simulink model "CryoDetMultiChan_CMB"  (R2016b)
settings: Solver=ode45  StartTime=0.0  StopTime=1000e-6  MaxStep=Tclk/4  RelTol=1e-3
values from neighbouring files (symbols this model uses):
  ds_axi = 16    [setupCryoFPGA_CMB.m]
  Fclk = Fadc    (= 307200000)    [setupCryoFPGA.m]    (also in setupCryoFPGA_CMB.m; setupCryoFPGAorig.m = 312500000)
  notch = tf( [1 a*wNotch/Q wNotch^2], [1 wNotch/Q wNotch^2])    [setupCryoFPGA.m]    (also in setupCryoFPGA_CMB.m; setupCryoFPGAorig.m)
  notch2 = tf( [1 a*wNotch/Q wNotch^2], [1 wNotch/Q wNotch^2])    [setupCryoFPGA.m]    (also in setupCryoFPGA_CMB.m; setupCryoFPGAorig.m)
  notch3 = tf( [1 a*wNotch/Q wNotch^2], [1 wNotch/Q wNotch^2])    [setupCryoFPGA.m]    (also in setupCryoFPGA_CMB.m; setupCryoFPGAorig.m)
  notch4 = tf( [1 a*wNotch/Q wNotch^2], [1 wNotch/Q wNotch^2])    [setupCryoFPGA.m]    (also in setupCryoFPGA_CMB.m; setupCryoFPGAorig.m)
  Tclk = 1/Fclk    (= 3.25520833333e-09)    [setupCryoFPGA.m]    (also in setupCryoFPGA_CMB.m; setupCryoFPGAorig.m = 3.2e-09)
  Ts = 1/Fadc    (= 3.25520833333e-09)    [setupCryoFPGA.m]    (also in setupCryoFPGA_CMB.m; setupCryoFPGAorig.m = 3.2e-09)
undefined symbols (not defined in the file or in its folder): AXI4, i, Lite, xlipgetpartsetting
libraries: xbsIndex_r4 x2077, CryoDetLib x32, hdlsllib x6, simulink x3
(part 6 of 15)

== system CryoDetMultiChan_CMB/DspCore/Status & Debug/DownSample ==
  note: DownSample with rate change given by Naxi
  In : Inport
  Down Sample : xbsIndex_r4/Down Sample  sample_ratio=Naxi  sample_phase="Last Value of Frame  (most efficient)"  en=off  rst=off  latency=1  dbl_ovrd=off  block_type=dsamp
  Register : xbsIndex_r4/Register  init=0  rst=off  en=off  dbl_ovrd=off  block_type=register
  Register1 : xbsIndex_r4/Register  init=0  rst=off  en=off  dbl_ovrd=off  block_type=register
  Out : Outport
  wires:
  Register1/1 -> Out/1
  Down Sample/1 -> Register/1
  In/1 -> Down Sample/1
  Register/1 -> Register1/1

== system CryoDetMultiChan_CMB/DspCore/Status & Debug/DownSample1 ==
  note: DownSample with rate change given by Naxi
  In : Inport
  Down Sample : xbsIndex_r4/Down Sample  sample_ratio=Naxi  sample_phase="Last Value of Frame  (most efficient)"  en=off  rst=off  latency=1  dbl_ovrd=off  block_type=dsamp
  Register : xbsIndex_r4/Register  init=0  rst=off  en=off  dbl_ovrd=off  block_type=register
  Register1 : xbsIndex_r4/Register  init=0  rst=off  en=off  dbl_ovrd=off  block_type=register
  Out : Outport
  wires:
  Register1/1 -> Out/1
  Down Sample/1 -> Register/1
  In/1 -> Down Sample/1
  Register/1 -> Register1/1

== system CryoDetMultiChan_CMB/DspCore/Status & Debug/DownSample10 ==
  note: DownSample with rate change given by Naxi
  In : Inport
  Down Sample : xbsIndex_r4/Down Sample  sample_ratio=Naxi  sample_phase="Last Value of Frame  (most efficient)"  en=off  rst=off  latency=1  dbl_ovrd=off  block_type=dsamp
  Register : xbsIndex_r4/Register  init=0  rst=off  en=off  dbl_ovrd=off  block_type=register
  Register1 : xbsIndex_r4/Register  init=0  rst=off  en=off  dbl_ovrd=off  block_type=register
  Out : Outport
  wires:
  Register1/1 -> Out/1
  Down Sample/1 -> Register/1
  In/1 -> Down Sample/1
  Register/1 -> Register1/1

== system CryoDetMultiChan_CMB/DspCore/Status & Debug/DownSample11 ==
  note: DownSample with rate change given by Naxi
  In : Inport
  Down Sample : xbsIndex_r4/Down Sample  sample_ratio=Naxi  sample_phase="Last Value of Frame  (most efficient)"  en=off  rst=off  latency=1  dbl_ovrd=off  block_type=dsamp
  Register : xbsIndex_r4/Register  init=0  rst=off  en=off  dbl_ovrd=off  block_type=register
  Register1 : xbsIndex_r4/Register  init=0  rst=off  en=off  dbl_ovrd=off  block_type=register
  Out : Outport
  wires:
  Register1/1 -> Out/1
  Down Sample/1 -> Register/1
  In/1 -> Down Sample/1
  Register/1 -> Register1/1

== system CryoDetMultiChan_CMB/DspCore/Status & Debug/DownSample12 ==
  note: DownSample with rate change given by Naxi
  In : Inport
  Down Sample : xbsIndex_r4/Down Sample  sample_ratio=Naxi  sample_phase="Last Value of Frame  (most efficient)"  en=off  rst=off  latency=1  dbl_ovrd=off  block_type=dsamp
  Register : xbsIndex_r4/Register  init=0  rst=off  en=off  dbl_ovrd=off  block_type=register
  Register1 : xbsIndex_r4/Register  init=0  rst=off  en=off  dbl_ovrd=off  block_type=register
  Out : Outport
  wires:
  Register1/1 -> Out/1
  Down Sample/1 -> Register/1
  In/1 -> Down Sample/1
  Register/1 -> Register1/1

== system CryoDetMultiChan_CMB/DspCore/Status & Debug/DownSample13 ==
  note: DownSample with rate change given by Naxi
  In : Inport
  Down Sample : xbsIndex_r4/Down Sample  sample_ratio=Naxi  sample_phase="Last Value of Frame  (most efficient)"  en=off  rst=off  latency=1  dbl_ovrd=off  block_type=dsamp
  Register : xbsIndex_r4/Register  init=0  rst=off  en=off  dbl_ovrd=off  block_type=register
  Register1 : xbsIndex_r4/Register  init=0  rst=off  en=off  dbl_ovrd=off  block_type=register
  Out : Outport
  wires:
  Register1/1 -> Out/1
  Down Sample/1 -> Register/1
  In/1 -> Down Sample/1
  Register/1 -> Register1/1

== system CryoDetMultiChan_CMB/DspCore/Status & Debug/DownSample14 ==
  note: DownSample with rate change given by Naxi
  In : Inport
  Down Sample : xbsIndex_r4/Down Sample  sample_ratio=Naxi  sample_phase="Last Value of Frame  (most efficient)"  en=off  rst=off  latency=1  dbl_ovrd=off  block_type=dsamp
  Register : xbsIndex_r4/Register  init=0  rst=off  en=off  dbl_ovrd=off  block_type=register
  Register1 : xbsIndex_r4/Register  init=0  rst=off  en=off  dbl_ovrd=off  block_type=register
  Out : Outport
  wires:
  Register1/1 -> Out/1
  Down Sample/1 -> Register/1
  In/1 -> Down Sample/1
  Register/1 -> Register1/1

== system CryoDetMultiChan_CMB/DspCore/Status & Debug/DownSample15 ==
  note: DownSample with rate change given by Naxi
  In : Inport
  Down Sample : xbsIndex_r4/Down Sample  sample_ratio=Naxi  sample_phase="Last Value of Frame  (most efficient)"  en=off  rst=off  latency=1  dbl_ovrd=off  block_type=dsamp
  Register : xbsIndex_r4/Register  init=0  rst=off  en=off  dbl_ovrd=off  block_type=register
  Register1 : xbsIndex_r4/Register  init=0  rst=off  en=off  dbl_ovrd=off  block_type=register
  Out : Outport
  wires:
  Register1/1 -> Out/1
  Down Sample/1 -> Register/1
  In/1 -> Down Sample/1
  Register/1 -> Register1/1

== system CryoDetMultiChan_CMB/DspCore/Status & Debug/DownSample16 ==
  note: DownSample with rate change given by Naxi
  In : Inport
  Down Sample : xbsIndex_r4/Down Sample  sample_ratio=Naxi  sample_phase="Last Value of Frame  (most efficient)"  en=off  rst=off  latency=1  dbl_ovrd=off  block_type=dsamp
  Register : xbsIndex_r4/Register  init=0  rst=off  en=off  dbl_ovrd=off  block_type=register
  Register1 : xbsIndex_r4/Register  init=0  rst=off  en=off  dbl_ovrd=off  block_type=register
  Out : Outport
  wires:
  Register1/1 -> Out/1
  Down Sample/1 -> Register/1
  In/1 -> Down Sample/1
  Register/1 -> Register1/1

== system CryoDetMultiChan_CMB/DspCore/Status & Debug/DownSample17 ==
  note: DownSample with rate change given by Naxi
  In : Inport
  Down Sample : xbsIndex_r4/Down Sample  sample_ratio=Naxi  sample_phase="Last Value of Frame  (most efficient)"  en=off  rst=off  latency=1  dbl_ovrd=off  block_type=dsamp
  Register : xbsIndex_r4/Register  init=0  rst=off  en=off  dbl_ovrd=off  block_type=register
  Register1 : xbsIndex_r4/Register  init=0  rst=off  en=off  dbl_ovrd=off  block_type=register
  Out : Outport
  wires:
  Register1/1 -> Out/1
  Down Sample/1 -> Register/1
  In/1 -> Down Sample/1
  Register/1 -> Register1/1

== system CryoDetMultiChan_CMB/DspCore/Status & Debug/DownSample18 ==
  note: DownSample with rate change given by Naxi
  In : Inport
  Down Sample : xbsIndex_r4/Down Sample  sample_ratio=Naxi  sample_phase="Last Value of Frame  (most efficient)"  en=off  rst=off  latency=1  dbl_ovrd=off  block_type=dsamp
  Register : xbsIndex_r4/Register  init=0  rst=off  en=off  dbl_ovrd=off  block_type=register
  Register1 : xbsIndex_r4/Register  init=0  rst=off  en=off  dbl_ovrd=off  block_type=register
  Out : Outport
  wires:
  Register1/1 -> Out/1
  Down Sample/1 -> Register/1
  In/1 -> Down Sample/1
  Register/1 -> Register1/1

== system CryoDetMultiChan_CMB/DspCore/Status & Debug/DownSample19 ==
  note: DownSample with rate change given by Naxi
  In : Inport
  Down Sample : xbsIndex_r4/Down Sample  sample_ratio=Naxi  sample_phase="Last Value of Frame  (most efficient)"  en=off  rst=off  latency=1  dbl_ovrd=off  block_type=dsamp
  Register : xbsIndex_r4/Register  init=0  rst=off  en=off  dbl_ovrd=off  block_type=register
  Register1 : xbsIndex_r4/Register  init=0  rst=off  en=off  dbl_ovrd=off  block_type=register
  Out : Outport
  wires:
  Register1/1 -> Out/1
  Down Sample/1 -> Register/1
  In/1 -> Down Sample/1
  Register/1 -> Register1/1

== system CryoDetMultiChan_CMB/DspCore/Status & Debug/DownSample2 ==
  note: DownSample with rate change given by Naxi
  In : Inport
  Down Sample : xbsIndex_r4/Down Sample  sample_ratio=Naxi  sample_phase="Last Value of Frame  (most efficient)"  en=off  rst=off  latency=1  dbl_ovrd=off  block_type=dsamp
  Register : xbsIndex_r4/Register  init=0  rst=off  en=off  dbl_ovrd=off  block_type=register
  Register1 : xbsIndex_r4/Register  init=0  rst=off  en=off  dbl_ovrd=off  block_type=register
  Out : Outport
  wires:
  Register1/1 -> Out/1
  Down Sample/1 -> Register/1
  In/1 -> Down Sample/1
  Register/1 -> Register1/1

== system CryoDetMultiChan_CMB/DspCore/Status & Debug/DownSample20 ==
  note: DownSample with rate change given by Naxi
  In : Inport
  Down Sample : xbsIndex_r4/Down Sample  sample_ratio=Naxi  sample_phase="Last Value of Frame  (most efficient)"  en=off  rst=off  latency=1  dbl_ovrd=off  block_type=dsamp
  Register : xbsIndex_r4/Register  init=0  rst=off  en=off  dbl_ovrd=off  block_type=register
  Register1 : xbsIndex_r4/Register  init=0  rst=off  en=off  dbl_ovrd=off  block_type=register
  Out : Outport
  wires:
  Register1/1 -> Out/1
  Down Sample/1 -> Register/1
  In/1 -> Down Sample/1
  Register/1 -> Register1/1

== system CryoDetMultiChan_CMB/DspCore/Status & Debug/DownSample21 ==
  note: DownSample with rate change given by Naxi
  In : Inport
  Down Sample : xbsIndex_r4/Down Sample  sample_ratio=Naxi  sample_phase="Last Value of Frame  (most efficient)"  en=off  rst=off  latency=1  dbl_ovrd=off  block_type=dsamp
  Register : xbsIndex_r4/Register  init=0  rst=off  en=off  dbl_ovrd=off  block_type=register
  Register1 : xbsIndex_r4/Register  init=0  rst=off  en=off  dbl_ovrd=off  block_type=register
  Out : Outport
  wires:
  Register1/1 -> Out/1
  Down Sample/1 -> Register/1
  In/1 -> Down Sample/1
  Register/1 -> Register1/1

== system CryoDetMultiChan_CMB/DspCore/Status & Debug/DownSample22 ==
  note: DownSample with rate change given by Naxi
  In : Inport
  Down Sample : xbsIndex_r4/Down Sample  sample_ratio=Naxi  sample_phase="Last Value of Frame  (most efficient)"  en=off  rst=off  latency=1  dbl_ovrd=off  block_type=dsamp
  Register : xbsIndex_r4/Register  init=0  rst=off  en=off  dbl_ovrd=off  block_type=register
  Register1 : xbsIndex_r4/Register  init=0  rst=off  en=off  dbl_ovrd=off  block_type=register
  Out : Outport
  wires:
  Register1/1 -> Out/1
  Down Sample/1 -> Register/1
  In/1 -> Down Sample/1
  Register/1 -> Register1/1

== system CryoDetMultiChan_CMB/DspCore/Status & Debug/DownSample23 ==
  note: DownSample with rate change given by Naxi
  In : Inport
  Down Sample : xbsIndex_r4/Down Sample  sample_ratio=Naxi  sample_phase="Last Value of Frame  (most efficient)"  en=off  rst=off  latency=1  dbl_ovrd=off  block_type=dsamp
  Register : xbsIndex_r4/Register  init=0  rst=off  en=off  dbl_ovrd=off  block_type=register
  Register1 : xbsIndex_r4/Register  init=0  rst=off  en=off  dbl_ovrd=off  block_type=register
  Out : Outport
  wires:
  Register1/1 -> Out/1
  Down Sample/1 -> Register/1
  In/1 -> Down Sample/1
  Register/1 -> Register1/1

== system CryoDetMultiChan_CMB/DspCore/Status & Debug/DownSample24 ==
  note: DownSample with rate change given by Naxi
  In : Inport
  Down Sample : xbsIndex_r4/Down Sample  sample_ratio=Naxi  sample_phase="Last Value of Frame  (most efficient)"  en=off  rst=off  latency=1  dbl_ovrd=off  block_type=dsamp
  Register : xbsIndex_r4/Register  init=0  rst=off  en=off  dbl_ovrd=off  block_type=register
  Register1 : xbsIndex_r4/Register  init=0  rst=off  en=off  dbl_ovrd=off  block_type=register
  Out : Outport
  wires:
  Register1/1 -> Out/1
  Down Sample/1 -> Register/1
  In/1 -> Down Sample/1
  Register/1 -> Register1/1

== system CryoDetMultiChan_CMB/DspCore/Status & Debug/DownSample25 ==
  note: DownSample with rate change given by Naxi
  In : Inport
  Down Sample : xbsIndex_r4/Down Sample  sample_ratio=Naxi  sample_phase="Last Value of Frame  (most efficient)"  en=off  rst=off  latency=1  dbl_ovrd=off  block_type=dsamp
  Register : xbsIndex_r4/Register  init=0  rst=off  en=off  dbl_ovrd=off  block_type=register
  Register1 : xbsIndex_r4/Register  init=0  rst=off  en=off  dbl_ovrd=off  block_type=register
  Out : Outport
  wires:
  Register1/1 -> Out/1
  Down Sample/1 -> Register/1
  In/1 -> Down Sample/1
  Register/1 -> Register1/1

== system CryoDetMultiChan_CMB/DspCore/Status & Debug/DownSample26 ==
  note: DownSample with rate change given by Naxi
  In : Inport
  Down Sample : xbsIndex_r4/Down Sample  sample_ratio=Naxi  sample_phase="Last Value of Frame  (most efficient)"  en=off  rst=off  latency=1  dbl_ovrd=off  block_type=dsamp
  Register : xbsIndex_r4/Register  init=0  rst=off  en=off  dbl_ovrd=off  block_type=register
  Register1 : xbsIndex_r4/Register  init=0  rst=off  en=off  dbl_ovrd=off  block_type=register
  Out : Outport
  wires:
  Register1/1 -> Out/1
  Down Sample/1 -> Register/1
  In/1 -> Down Sample/1
  Register/1 -> Register1/1

== system CryoDetMultiChan_CMB/DspCore/Status & Debug/DownSample27 ==
  note: DownSample with rate change given by Naxi
  In : Inport
  Down Sample : xbsIndex_r4/Down Sample  sample_ratio=Naxi  sample_phase="Last Value of Frame  (most efficient)"  en=off  rst=off  latency=1  dbl_ovrd=off  block_type=dsamp
  Register : xbsIndex_r4/Register  init=0  rst=off  en=off  dbl_ovrd=off  block_type=register
  Register1 : xbsIndex_r4/Register  init=0  rst=off  en=off  dbl_ovrd=off  block_type=register
  Out : Outport
  wires:
  Register1/1 -> Out/1
  Down Sample/1 -> Register/1
  In/1 -> Down Sample/1
  Register/1 -> Register1/1

== system CryoDetMultiChan_CMB/DspCore/Status & Debug/DownSample28 ==
  note: DownSample with rate change given by Naxi
  In : Inport
  Down Sample : xbsIndex_r4/Down Sample  sample_ratio=Naxi  sample_phase="Last Value of Frame  (most efficient)"  en=off  rst=off  latency=1  dbl_ovrd=off  block_type=dsamp
  Register : xbsIndex_r4/Register  init=0  rst=off  en=off  dbl_ovrd=off  block_type=register
  Register1 : xbsIndex_r4/Register  init=0  rst=off  en=off  dbl_ovrd=off  block_type=register
  Out : Outport
  wires:
  Register1/1 -> Out/1
  Down Sample/1 -> Register/1
  In/1 -> Down Sample/1
  Register/1 -> Register1/1

== system CryoDetMultiChan_CMB/DspCore/Status & Debug/DownSample29 ==
  note: DownSample with rate change given by Naxi
  In : Inport
  Down Sample : xbsIndex_r4/Down Sample  sample_ratio=Naxi  sample_phase="Last Value of Frame  (most efficient)"  en=off  rst=off  latency=1  dbl_ovrd=off  block_type=dsamp
  Register : xbsIndex_r4/Register  init=0  rst=off  en=off  dbl_ovrd=off  block_type=register
  Register1 : xbsIndex_r4/Register  init=0  rst=off  en=off  dbl_ovrd=off  block_type=register
  Out : Outport
  wires:
  Register1/1 -> Out/1
  Down Sample/1 -> Register/1
  In/1 -> Down Sample/1
  Register/1 -> Register1/1

== system CryoDetMultiChan_CMB/DspCore/Status & Debug/DownSample3 ==
  note: DownSample with rate change given by Naxi
  In : Inport
  Down Sample : xbsIndex_r4/Down Sample  sample_ratio=Naxi  sample_phase="Last Value of Frame  (most efficient)"  en=off  rst=off  latency=1  dbl_ovrd=off  block_type=dsamp
  Register : xbsIndex_r4/Register  init=0  rst=off  en=off  dbl_ovrd=off  block_type=register
  Register1 : xbsIndex_r4/Register  init=0  rst=off  en=off  dbl_ovrd=off  block_type=register
  Out : Outport
  wires:
  Register1/1 -> Out/1
  Down Sample/1 -> Register/1
  In/1 -> Down Sample/1
  Register/1 -> Register1/1

== system CryoDetMultiChan_CMB/DspCore/Status & Debug/DownSample30 ==
  note: DownSample with rate change given by Naxi
  In : Inport
  Down Sample : xbsIndex_r4/Down Sample  sample_ratio=Naxi  sample_phase="Last Value of Frame  (most efficient)"  en=off  rst=off  latency=1  dbl_ovrd=off  block_type=dsamp
  Register : xbsIndex_r4/Register  init=0  rst=off  en=off  dbl_ovrd=off  block_type=register
  Register1 : xbsIndex_r4/Register  init=0  rst=off  en=off  dbl_ovrd=off  block_type=register
  Out : Outport
  wires:
  Register1/1 -> Out/1
  Down Sample/1 -> Register/1
  In/1 -> Down Sample/1
  Register/1 -> Register1/1

== system CryoDetMultiChan_CMB/DspCore/Status & Debug/DownSample31 ==
  note: DownSample with rate change given by Naxi
  In : Inport
  Down Sample : xbsIndex_r4/Down Sample  sample_ratio=Naxi  sample_phase="Last Value of Frame  (most efficient)"  en=off  rst=off  latency=1  dbl_ovrd=off  block_type=dsamp
  Register : xbsIndex_r4/Register  init=0  rst=off  en=off  dbl_ovrd=off  block_type=register
  Register1 : xbsIndex_r4/Register  init=0  rst=off  en=off  dbl_ovrd=off  block_type=register
  Out : Outport
  wires:
  Register1/1 -> Out/1
  Down Sample/1 -> Register/1
  In/1 -> Down Sample/1
  Register/1 -> Register1/1

== system CryoDetMultiChan_CMB/DspCore/Status & Debug/DownSample32 ==
  note: DownSample with rate change given by Naxi
  In : Inport
  Down Sample : xbsIndex_r4/Down Sample  sample_ratio=Naxi  sample_phase="Last Value of Frame  (most efficient)"  en=off  rst=off  latency=1  dbl_ovrd=off  block_type=dsamp
  Register : xbsIndex_r4/Register  init=0  rst=off  en=off  dbl_ovrd=off  block_type=register
  Register1 : xbsIndex_r4/Register  init=0  rst=off  en=off  dbl_ovrd=off  block_type=register
  Out : Outport
  wires:
  Register1/1 -> Out/1
  Down Sample/1 -> Register/1
  In/1 -> Down Sample/1
  Register/1 -> Register1/1

== system CryoDetMultiChan_CMB/DspCore/Status & Debug/DownSample33 ==
  note: DownSample with rate change given by Naxi
  In : Inport
  Down Sample : xbsIndex_r4/Down Sample  sample_ratio=Naxi  sample_phase="Last Value of Frame  (most efficient)"  en=off  rst=off  latency=1  dbl_ovrd=off  block_type=dsamp
  Register : xbsIndex_r4/Register  init=0  rst=off  en=off  dbl_ovrd=off  block_type=register
  Register1 : xbsIndex_r4/Register  init=0  rst=off  en=off  dbl_ovrd=off  block_type=register
  Out : Outport
  wires:
  Register1/1 -> Out/1
  Down Sample/1 -> Register/1
  In/1 -> Down Sample/1
  Register/1 -> Register1/1

== system CryoDetMultiChan_CMB/DspCore/Status & Debug/DownSample34 ==
  note: DownSample with rate change given by Naxi
  In : Inport
  Down Sample : xbsIndex_r4/Down Sample  sample_ratio=Naxi  sample_phase="Last Value of Frame  (most efficient)"  en=off  rst=off  latency=1  dbl_ovrd=off  block_type=dsamp
  Register : xbsIndex_r4/Register  init=0  rst=off  en=off  dbl_ovrd=off  block_type=register
  Register1 : xbsIndex_r4/Register  init=0  rst=off  en=off  dbl_ovrd=off  block_type=register
  Out : Outport
  wires:
  Register1/1 -> Out/1
  Down Sample/1 -> Register/1
  In/1 -> Down Sample/1
  Register/1 -> Register1/1

== system CryoDetMultiChan_CMB/DspCore/Status & Debug/DownSample35 ==
  note: DownSample with rate change given by Naxi
  In : Inport
  Down Sample : xbsIndex_r4/Down Sample  sample_ratio=Naxi  sample_phase="Last Value of Frame  (most efficient)"  en=off  rst=off  latency=1  dbl_ovrd=off  block_type=dsamp
  Register : xbsIndex_r4/Register  init=0  rst=off  en=off  dbl_ovrd=off  block_type=register
  Register1 : xbsIndex_r4/Register  init=0  rst=off  en=off  dbl_ovrd=off  block_type=register
  Out : Outport
  wires:
  Register1/1 -> Out/1
  Down Sample/1 -> Register/1
  In/1 -> Down Sample/1
  Register/1 -> Register1/1

== system CryoDetMultiChan_CMB/DspCore/Status & Debug/DownSample36 ==
  note: DownSample with rate change given by Naxi
  In : Inport
  Down Sample : xbsIndex_r4/Down Sample  sample_ratio=Naxi  sample_phase="Last Value of Frame  (most efficient)"  en=off  rst=off  latency=1  dbl_ovrd=off  block_type=dsamp
  Register : xbsIndex_r4/Register  init=0  rst=off  en=off  dbl_ovrd=off  block_type=register
  Register1 : xbsIndex_r4/Register  init=0  rst=off  en=off  dbl_ovrd=off  block_type=register
  Out : Outport
  wires:
  Register1/1 -> Out/1
  Down Sample/1 -> Register/1
  In/1 -> Down Sample/1
  Register/1 -> Register1/1

== system CryoDetMultiChan_CMB/DspCore/Status & Debug/DownSample37 ==
  note: DownSample with rate change given by Naxi
  In : Inport
  Down Sample : xbsIndex_r4/Down Sample  sample_ratio=Naxi  sample_phase="Last Value of Frame  (most efficient)"  en=off  rst=off  latency=1  dbl_ovrd=off  block_type=dsamp
  Register : xbsIndex_r4/Register  init=0  rst=off  en=off  dbl_ovrd=off  block_type=register
  Register1 : xbsIndex_r4/Register  init=0  rst=off  en=off  dbl_ovrd=off  block_type=register
  Out : Outport
  wires:
  Register1/1 -> Out/1
  Down Sample/1 -> Register/1
  In/1 -> Down Sample/1
  Register/1 -> Register1/1

== system CryoDetMultiChan_CMB/DspCore/Status & Debug/DownSample38 ==
  note: DownSample with rate change given by Naxi
  In : Inport
  Down Sample : xbsIndex_r4/Down Sample  sample_ratio=Naxi  sample_phase="Last Value of Frame  (most efficient)"  en=off  rst=off  latency=1  dbl_ovrd=off  block_type=dsamp
  Register : xbsIndex_r4/Register  init=0  rst=off  en=off  dbl_ovrd=off  block_type=register
  Register1 : xbsIndex_r4/Register  init=0  rst=off  en=off  dbl_ovrd=off  block_type=register
  Out : Outport
  wires:
  Register1/1 -> Out/1
  Down Sample/1 -> Register/1
  In/1 -> Down Sample/1
  Register/1 -> Register1/1

== system CryoDetMultiChan_CMB/DspCore/Status & Debug/DownSample39 ==
  note: DownSample with rate change given by Naxi
  In : Inport
  Down Sample : xbsIndex_r4/Down Sample  sample_ratio=Naxi  sample_phase="Last Value of Frame  (most efficient)"  en=off  rst=off  latency=1  dbl_ovrd=off  block_type=dsamp
  Register : xbsIndex_r4/Register  init=0  rst=off  en=off  dbl_ovrd=off  block_type=register
  Register1 : xbsIndex_r4/Register  init=0  rst=off  en=off  dbl_ovrd=off  block_type=register
  Out : Outport
  wires:
  Register1/1 -> Out/1
  Down Sample/1 -> Register/1
  In/1 -> Down Sample/1
  Register/1 -> Register1/1

== system CryoDetMultiChan_CMB/DspCore/Status & Debug/DownSample4 ==
  note: DownSample with rate change given by Naxi
  In : Inport
  Down Sample : xbsIndex_r4/Down Sample  sample_ratio=Naxi  sample_phase="Last Value of Frame  (most efficient)"  en=off  rst=off  latency=1  dbl_ovrd=off  block_type=dsamp
  Register : xbsIndex_r4/Register  init=0  rst=off  en=off  dbl_ovrd=off  block_type=register
  Register1 : xbsIndex_r4/Register  init=0  rst=off  en=off  dbl_ovrd=off  block_type=register
  Out : Outport
  wires:
  Register1/1 -> Out/1
  Down Sample/1 -> Register/1
  In/1 -> Down Sample/1
  Register/1 -> Register1/1

== system CryoDetMultiChan_CMB/DspCore/Status & Debug/DownSample40 ==
  note: DownSample with rate change given by Naxi
  In : Inport
  Down Sample : xbsIndex_r4/Down Sample  sample_ratio=Naxi  sample_phase="Last Value of Frame  (most efficient)"  en=off  rst=off  latency=1  dbl_ovrd=off  block_type=dsamp
  Register : xbsIndex_r4/Register  init=0  rst=off  en=off  dbl_ovrd=off  block_type=register
  Register1 : xbsIndex_r4/Register  init=0  rst=off  en=off  dbl_ovrd=off  block_type=register
  Out : Outport
  wires:
  Register1/1 -> Out/1
  Down Sample/1 -> Register/1
  In/1 -> Down Sample/1
  Register/1 -> Register1/1

== system CryoDetMultiChan_CMB/DspCore/Status & Debug/DownSample41 ==
  note: DownSample with rate change given by Naxi
  In : Inport
  Down Sample : xbsIndex_r4/Down Sample  sample_ratio=Naxi  sample_phase="Last Value of Frame  (most efficient)"  en=off  rst=off  latency=1  dbl_ovrd=off  block_type=dsamp
  Register : xbsIndex_r4/Register  init=0  rst=off  en=off  dbl_ovrd=off  block_type=register
  Register1 : xbsIndex_r4/Register  init=0  rst=off  en=off  dbl_ovrd=off  block_type=register
  Out : Outport
  wires:
  Register1/1 -> Out/1
  Down Sample/1 -> Register/1
  In/1 -> Down Sample/1
  Register/1 -> Register1/1

== system CryoDetMultiChan_CMB/DspCore/Status & Debug/DownSample5 ==
  note: DownSample with rate change given by Naxi
  In : Inport
  Down Sample : xbsIndex_r4/Down Sample  sample_ratio=Naxi  sample_phase="Last Value of Frame  (most efficient)"  en=off  rst=off  latency=1  dbl_ovrd=off  block_type=dsamp
  Register : xbsIndex_r4/Register  init=0  rst=off  en=off  dbl_ovrd=off  block_type=register
  Register1 : xbsIndex_r4/Register  init=0  rst=off  en=off  dbl_ovrd=off  block_type=register
  Out : Outport
  wires:
  Register1/1 -> Out/1
  Down Sample/1 -> Register/1
  In/1 -> Down Sample/1
  Register/1 -> Register1/1

== system CryoDetMultiChan_CMB/DspCore/Status & Debug/DownSample6 ==
  note: DownSample with rate change given by Naxi
  In : Inport
  Down Sample : xbsIndex_r4/Down Sample  sample_ratio=Naxi  sample_phase="Last Value of Frame  (most efficient)"  en=off  rst=off  latency=1  dbl_ovrd=off  block_type=dsamp
  Register : xbsIndex_r4/Register  init=0  rst=off  en=off  dbl_ovrd=off  block_type=register
  Register1 : xbsIndex_r4/Register  init=0  rst=off  en=off  dbl_ovrd=off  block_type=register
  Out : Outport
  wires:
  Register1/1 -> Out/1
  Down Sample/1 -> Register/1
  In/1 -> Down Sample/1
  Register/1 -> Register1/1

== system CryoDetMultiChan_CMB/DspCore/Status & Debug/DownSample7 ==
  note: DownSample with rate change given by Naxi
  In : Inport
  Down Sample : xbsIndex_r4/Down Sample  sample_ratio=Naxi  sample_phase="Last Value of Frame  (most efficient)"  en=off  rst=off  latency=1  dbl_ovrd=off  block_type=dsamp
  Register : xbsIndex_r4/Register  init=0  rst=off  en=off  dbl_ovrd=off  block_type=register
  Register1 : xbsIndex_r4/Register  init=0  rst=off  en=off  dbl_ovrd=off  block_type=register
  Out : Outport
  wires:
  Register1/1 -> Out/1
  Down Sample/1 -> Register/1
  In/1 -> Down Sample/1
  Register/1 -> Register1/1

== system CryoDetMultiChan_CMB/DspCore/Status & Debug/DownSample8 ==
  note: DownSample with rate change given by Naxi
  In : Inport
  Down Sample : xbsIndex_r4/Down Sample  sample_ratio=Naxi  sample_phase="Last Value of Frame  (most efficient)"  en=off  rst=off  latency=1  dbl_ovrd=off  block_type=dsamp
  Register : xbsIndex_r4/Register  init=0  rst=off  en=off  dbl_ovrd=off  block_type=register
  Register1 : xbsIndex_r4/Register  init=0  rst=off  en=off  dbl_ovrd=off  block_type=register
  Out : Outport
  wires:
  Register1/1 -> Out/1
  Down Sample/1 -> Register/1
  In/1 -> Down Sample/1
  Register/1 -> Register1/1

== system CryoDetMultiChan_CMB/DspCore/Status & Debug/DownSample9 ==
  note: DownSample with rate change given by Naxi
  In : Inport
  Down Sample : xbsIndex_r4/Down Sample  sample_ratio=Naxi  sample_phase="Last Value of Frame  (most efficient)"  en=off  rst=off  latency=1  dbl_ovrd=off  block_type=dsamp
  Register : xbsIndex_r4/Register  init=0  rst=off  en=off  dbl_ovrd=off  block_type=register
  Register1 : xbsIndex_r4/Register  init=0  rst=off  en=off  dbl_ovrd=off  block_type=register
  Out : Outport
  wires:
  Register1/1 -> Out/1
  Down Sample/1 -> Register/1
  In/1 -> Down Sample/1
  Register/1 -> Register1/1

== system CryoDetMultiChan_CMB/DspCore/FTA_Ch0/SixteenLineUDC 0/DAC Sum1 ==
  note: Sum I0, Q0, I1, Q1 across all 16 input channels
  note: Changed from 12 channel to 16 channels 8Sept2017
  note: DAC Sum
      |
      | Sums the I & Q portions of the DAC and DAC + phi words from each channel into four streams of DAC_Q, DAC_I, DACp_Q, DACp_I (DACp = DAC + phi)
  In1 : Inport
  In2 : Inport  Port=2
  In3 : Inport  Port=3
  In4 : Inport  Port=4
  In5 : Inport  Port=5
  In6 : Inport  Port=6
  In7 : Inport  Port=7
  In8 : Inport  Port=8
  In9 : Inport  Port=9
  In10 : Inport  Port=10
  In11 : Inport  Port=11
  In12 : Inport  Port=12
  In13 : Inport  Port=13
  In14 : Inport  Port=14
  In15 : Inport  Port=15
  In16 : Inport  Port=16
  Bus Creator : BusCreator  Inputs=4
  Bus Creator1 : BusCreator  Inputs=16
  DAC UC I sum : Subsystem
  DAC UC Q sum : Subsystem
  DAC UC Qi sum : Subsystem
  DAC UC Qp sum : Subsystem
  Out1 : Outport
  wires:
  In3/1 -> Bus Creator1/3
  In4/1 -> Bus Creator1/4
  In5/1 -> Bus Creator1/5
  In6/1 -> Bus Creator1/6
  In7/1 -> Bus Creator1/7
  In8/1 -> Bus Creator1/8
  In9/1 -> Bus Creator1/9
  In11/1 -> Bus Creator1/11
  In12/1 -> Bus Creator1/12
  In13/1 -> Bus Creator1/13
  In14/1 -> Bus Creator1/14
  In15/1 -> Bus Creator1/15
  In16/1 -> Bus Creator1/16
  In2/1 -> Bus Creator1/2
  In1/1 -> Bus Creator1/1
  In10/1 -> Bus Creator1/10
  Bus Creator1/1 -> DAC UC Qi sum/1(In1), DAC UC Qp sum/1(In1), DAC UC Q sum/1(In1), DAC UC I sum/1(In1)
  DAC UC Q sum/1(Out1) -> Bus Creator/1  "Q sum"
  DAC UC I sum/1(Out1) -> Bus Creator/2  "I sum"
  DAC UC Qp sum/1(Out1) -> Bus Creator/3  "Qp sum"
  DAC UC Qi sum/1(Out1) -> Bus Creator/4  "Ip sum"
  Bus Creator/1 -> Out1/1

== system CryoDetMultiChan_CMB/DspCore/FTA_Ch0/SixteenLineUDC 0/DC_decimate ==
  note: When data not available send Ch 16 as
      | a kludge for now
      | eta and dF shouod look at tvalid instead
  note: tvalid
  note: Ref-
  note: dec_ref_IQ0
  note: dec_sig_IQ0
  note: for synchonization/channel identification:
      | read input channel number  from input multiplexer (delayed by latency of complex multiplier)
      | as latched by data_tlast at input of CIC to get channel number offset at output of CIC wrt to data_tuser_chan_out
  note: Every clock another lines presents 4 components to the sideband demodulator
  note: signal
      | central line
  note: Signal
  note: Reference
  note: reference
      | central line
  note: Channel #
  note: Sig_Q
  note: Sig_I
  note: Ref_Q
  note: REf_I
  note: dec_Sig_Q
  note: dec_Sig_I
  note: dec_Ref_Q
  note: dec_Ref_I
  note: Channel #
  In1 : Inport
  1c demod Scope : Scope  NumInputPorts=3
  Bus Creator : BusCreator  Inputs=2
  Bus Creator1 : BusCreator  Inputs=2
  CIC Compiler 4.0 {,1,6..7} (4 alike) : xbsIndex_r4/CIC Compiler 4.0   filter_type=Decimation  number_of_stages=3  differential_delay=1  number_of_channels=16  sample_rate_changes=Fixed  fixed_or_initial_rate=16  minimum_rate=16  maximum_rate=16  ratespecification=Sample_Period  sampleperiod=1  hardwareoversamplingrate=1  quantization=Truncation  output_data_width=24  use_xtreme_dsp_slice=off  use_streaming_interface=off  has_aclken=off  has_aresetn=on  has_dout_tready=off  trim_axipin_name=on  gui_behaviour=Sysgen_GUI  input_data_width=18  ip_name=CIC Compiler  ip_version=4.0  dsptool_ready=true  wrapper_available=true  port_translation_map={ 'aclken' => 'en', 'aresetn' => 'rst' }  ipcore_xco_need_fpga_part=true  ipcore_verbose=false  block_type=cic_compiler_v4_0
  CIC reset : Subsystem
  Constant : xbsIndex_r4/Constant  const=1.0  gui_display_data_type=Boolean  arith_type=Boolean  n_bits=16  bin_pt=14  preci_type=Single  exp_width=8  frac_width=24  explicit_period=off  period=1  equ=P=C  opselect=C  inp2=PCIN>>17  opr=+  inp1=P  carry=CIN  dbl_ovrd=off  block_type=constant
  Constant1 : xbsIndex_r4/Constant  const=16  gui_display_data_type=Fixed-point  arith_type=Unsigned  n_bits=5  bin_pt=0  preci_type=Single  exp_width=8  frac_width=24  explicit_period=off  period=1  equ=P=C  opselect=C  inp2=PCIN>>17  opr=+  inp1=P  carry=CIN  dbl_ovrd=off  block_type=constant
  Constant4 : xbsIndex_r4/Constant  const=14  gui_display_data_type=Fixed-point  arith_type=Unsigned  n_bits=5  bin_pt=0  preci_type=Single  exp_width=8  frac_width=24  explicit_period=off  period=1  equ=P=C  opselect=C  inp2=PCIN>>17  opr=+  inp1=P  carry=CIN  dbl_ovrd=off  block_type=constant
  Delay{1..5} (5 alike) : xbsIndex_r4/Delay  rst=off  infoeditControl=Selection of Reset will increase slice count due to use of real FFs and instead of SRLs  en=off  latency=6  reg_retiming=off  dbl_ovrd=off  block_type=delay
  Delay6 : xbsIndex_r4/Delay  rst=off  infoeditControl=Selection of Reset will increase slice count due to use of real FFs and instead of SRLs  en=off  latency=4  reg_retiming=off  dbl_ovrd=off  block_type=delay
  Demux{,1,3..4} (4 alike) : Demux  Outputs=2
  Demux2 : Demux  Outputs=6
  Gateway Out{1..6} (6 alike) : xbsIndex_r4/Gateway Out  inherit_from_input=off  hdl_port=off  rows=1  columns=1  UseAsDAC=off  DACChannel='1'  interface=None  automatic_assignment=on  address_offset=hex2dec('00')  intf_name=''  intf_description=''  timing_constraint=None  locs_specified=off  LOCs={}  io_standard={}  block_type=gatewayout
  Mux{1..2,4,7..9} (6 alike) : Mux  Inputs=2
  Mux14 : xbsIndex_r4/Mux  inputs=2  en=off  latency=0  precision=Full  arith_type=Unsigned  n_bits=16  bin_pt=14  quantization=Truncate  overflow=Wrap  dbl_ovrd=off  block_type=mux
  Scale{1..2,7..8} (4 alike) : xbsIndex_r4/Scale  scale_factor=-12  dbl_ovrd=off  block_type=scale
  Scope : Scope  NumInputPorts=3
  dec_sig_ref : Outport
  wires:
  "CIC Compiler 4.0 "/3 -> Scale1/1
  Demux/1 -> Demux1/1
  Demux1/1 -> Delay2/1
  Demux1/2 -> Delay1/1
  Demux/2 -> Demux4/1
  CIC reset/2(tlast) -> Scope/1, "CIC Compiler 4.0 "/3, CIC Compiler 4.0 1/3, CIC Compiler 4.0 6/3, CIC Compiler 4.0 7/3  "tlast"
  CIC reset/1(notResetOut) -> CIC Compiler 4.0 1/4, CIC Compiler 4.0 6/4, CIC Compiler 4.0 7/4, "CIC Compiler 4.0 "/4
  In1/1 -> Demux3/1
  Demux3/2 -> Demux/1  "SIG_and_REF"
  Delay1/1 -> Scope/3, CIC Compiler 4.0 1/2
  Delay2/1 -> "CIC Compiler 4.0 "/2
  CIC Compiler 4.0 1/3 -> Scale2/1
  Demux4/1 -> Delay5/1
  Demux4/2 -> Delay4/1
  Constant/1 -> "CIC Compiler 4.0 "/1, CIC Compiler 4.0 1/1, CIC Compiler 4.0 6/1, CIC Compiler 4.0 7/1
  Delay4/1 -> CIC Compiler 4.0 7/2
  Delay5/1 -> CIC Compiler 4.0 6/2
  CIC Compiler 4.0 6/3 -> Scale7/1
  CIC Compiler 4.0 7/3 -> Scale8/1
  Delay3/1 -> Scope/2, CIC reset/2(Channel)
  Scale2/1 -> Mux1/2
  Scale1/1 -> Mux1/1
  Scale7/1 -> Mux4/1
  Scale8/1 -> Mux4/2
  Mux4/1 -> Mux2/2
  Mux1/1 -> Mux2/1
  Mux2/1 -> Bus Creator/2  "decSigandRef"
  Demux3/1 -> Delay6/1, Delay3/1  "channel"
  CIC Compiler 4.0 6/2 -> Bus Creator1/2, Mux14/1  "valid"
  Bus Creator1/1 -> Bus Creator/1  "chanAndTvalid"
  Bus Creator/1 -> Demux2/1, dec_sig_ref/1
  Demux2/1 -> Gateway Out3/1
  Demux2/2 -> Gateway Out4/1
  Demux2/3 -> Gateway Out5/1
  Demux2/4 -> Gateway Out6/1
  Gateway Out6/1 -> Mux8/2
  Gateway Out5/1 -> Mux8/1
  Gateway Out4/1 -> Mux7/2
  Gateway Out3/1 -> Mux7/1
  Mux7/1 -> 1c demod Scope/1
  Mux8/1 -> 1c demod Scope/2
  Demux2/6 -> Gateway Out2/1
  Gateway Out2/1 -> Mux9/2
  Gateway Out1/1 -> Mux9/1
  Demux2/5 -> Gateway Out1/1
  Mux9/1 -> 1c demod Scope/3
  Constant4/1 -> CIC reset/3(N-2)
  [fpgaReset] -> CIC reset/1(resetIn)
  Delay6/1 -> Mux14/3  "channel"
  Constant1/1 -> Mux14/2
  Mux14/1 -> Bus Creator1/1  "channel"

== system CryoDetMultiChan_CMB/DspCore/FTA_Ch0/SixteenLineUDC 0/Mux16X4 ==
  note: <09-25-2017 JED>: For Multi-Channel Version / Changed Channel Counter to 5b & make it roll over @ 31, changes channel bus to 5b
  note: Extract bits [3:0] here
  note: Channel Counter:
      | master sequence counter
  note: I think this will select a channel 1 or 2 ticks after it has updated,
      | which should work fine. But optimal would be to delay synch in by 15 ticks = N-1
  note: Channel ID
  note: Reference Q&I
  note: Signal Q&I
  note: Sixteen busses 4-wide each time-division multiplexed onto a 4-wide bus
  note: MUX16x4
      |
      | Performs the time-inerleaving of the ADC and Reference signals via a Mux structure, whose selection input is driven by a counter. The input data is assumed to be at the correct time relationship for mux'ing. Tjhe channel # is also forwarded with the output stream to tag the data.
  synch : Inport
  line0 : Inport  Port=2
  line1 : Inport  Port=3
  line2 : Inport  Port=4
  line3 : Inport  Port=5
  line4 : Inport  Port=6
  line5 : Inport  Port=7
  line6 : Inport  Port=8
  line7 : Inport  Port=9
  line8 : Inport  Port=10
  line9 : Inport  Port=11
  line10 : Inport  Port=12
  line11 : Inport  Port=13
  line12 : Inport  Port=14
  line13 : Inport  Port=15
  line14 : Inport  Port=16
  line15 : Inport  Port=17
  BitBasher : xbsIndex_r4/BitBasher  bitexpr=a={b[3:0]}  display_expr=off  sr_1=a  arith_type1=Unsigned  bin_pt1=0  sr_2=2  arith_type2=Unsigned  bin_pt2=0  sr_3=3  arith_type3=Unsigned  bin_pt3=0  sr_4=4  arith_type4=Unsigned  bin_pt4=0  dbl_ovrd=off  block_type=bitbasher
  Bus Creator{,1..3} (4 alike) : BusCreator  Inputs=2
  Counter : xbsIndex_r4/Counter  cnt_type=Count Limited  cnt_to=31  operation=Up  start_count=0  cnt_by_val=1  arith_type=Unsigned  n_bits=5  bin_pt=0  load_pin=off  rst=on  en=off  explicit_period=off  period=Tclk  use_behavioral_HDL=off  implementation=Fabric  dbl_ovrd=off  block_type=counter
  Delay1 : xbsIndex_r4/Delay  rst=off  infoeditControl=Selection of Reset will increase slice count due to use of real FFs and instead of SRLs  en=off  latency=1  reg_retiming=off  dbl_ovrd=off  block_type=delay
  Demux{,1..15} (16 alike) : Demux
  Gateway Out{3..6} (4 alike) : xbsIndex_r4/Gateway Out  inherit_from_input=off  hdl_port=off  rows=1  columns=1  UseAsDAC=off  DACChannel='1'  interface=None  automatic_assignment=on  address_offset=hex2dec('00')  intf_name=''  intf_description=''  timing_constraint=None  locs_specified=off  LOCs={}  io_standard={}  block_type=gatewayout
  Mux{,1..3} (4 alike) : xbsIndex_r4/Mux  inputs=16  en=off  latency=1  precision=Full  arith_type=Unsigned  n_bits=16  bin_pt=14  quantization=Truncate  overflow=Wrap  dbl_ovrd=off  block_type=mux
  Mux4 : Mux  Inputs=2
  Mux5 : Mux  Inputs=2
  Scope : Scope  NumInputPorts=3
  block downconverter Scope : Scope  NumInputPorts=3
  Out1 : Outport
  wires:
  line0/1 -> Demux/1
  line5/1 -> Demux6/1
  line4/1 -> Demux5/1
  line3/1 -> Demux4/1
  line2/1 -> Demux3/1
  line1/1 -> Demux1/1
  Demux/1 -> Mux/2
  Demux/2 -> Mux1/2
  Demux/3 -> Mux2/2
  Demux/4 -> Mux3/2
  Demux1/1 -> Mux/3
  Demux1/2 -> Mux1/3
  Demux1/3 -> Mux2/3
  Demux1/4 -> Mux3/3
  Demux3/1 -> Mux/4
  Demux3/2 -> Mux1/4
  Demux3/3 -> Mux2/4
  Demux3/4 -> Mux3/4
  Demux4/1 -> Mux/5
  Demux4/2 -> Mux1/5
  Demux4/3 -> Mux2/5
  Demux4/4 -> Mux3/5
  Demux5/1 -> Mux/6
  Demux5/2 -> Mux1/6
  Demux5/3 -> Mux2/6
  Demux5/4 -> Mux3/6
  Demux6/1 -> Mux/7
  Demux6/2 -> Mux1/7
  Demux6/3 -> Mux2/7
  Demux6/4 -> Mux3/7
  synch/1 -> Scope/3, Counter/1
  Mux/1 -> Gateway Out4/1, Bus Creator1/1  "sig_Q"
  Mux1/1 -> Gateway Out3/1, Bus Creator1/2  "sig_I"
  Mux2/1 -> Gateway Out6/1, Bus Creator2/1  "ref_Q"
  Mux3/1 -> Gateway Out5/1, Bus Creator2/2  "ref_I"
  Bus Creator1/1 -> Bus Creator3/1  "SignalQ&I"
  Bus Creator2/1 -> Bus Creator3/2  "ReferenceQ&I"
  Counter/1 -> Scope/1, BitBasher/1, Delay1/1
  Bus Creator3/1 -> Bus Creator/2  "Sig&Ref"
  Delay1/1 -> block downconverter Scope/3, Bus Creator/1  "channel"
  Bus Creator/1 -> Out1/1
  line8/1 -> Demux2/1
  line9/1 -> Demux7/1
  line10/1 -> Demux8/1
  line11/1 -> Demux9/1
  line12/1 -> Demux10/1
  line13/1 -> Demux11/1
  line7/1 -> Demux13/1
  line6/1 -> Demux12/1
  line14/1 -> Demux14/1
  line15/1 -> Demux15/1
  Demux14/3 -> Mux2/16
  Demux12/1 -> Mux/8
  Demux12/2 -> Mux1/8
  Demux12/3 -> Mux2/8
  Demux12/4 -> Mux3/8
  Demux13/1 -> Mux/9
  Demux13/2 -> Mux1/9
  Demux13/3 -> Mux2/9
  Demux13/4 -> Mux3/9
  Demux2/1 -> Mux/10
  Demux2/2 -> Mux1/10
  Demux2/3 -> Mux2/10
  Demux2/4 -> Mux3/10
  Demux7/1 -> Mux/11
  Demux7/2 -> Mux1/11
  Demux7/3 -> Mux2/11
  Demux7/4 -> Mux3/11
  Demux8/1 -> Mux/12
  Demux8/2 -> Mux1/12
  Demux8/3 -> Mux2/12
  Demux8/4 -> Mux3/12
  Demux9/1 -> Mux/13
  Demux9/2 -> Mux1/13
  Demux9/3 -> Mux2/13
  Demux9/4 -> Mux3/13
  Demux10/1 -> Mux/14
  Demux10/2 -> Mux1/14
  Demux10/3 -> Mux2/14
  Demux10/4 -> Mux3/14
  Demux11/1 -> Mux/15
  Demux11/2 -> Mux1/15
  Demux11/3 -> Mux2/15
  Demux11/4 -> Mux3/15
  Demux14/1 -> Mux/16
  Demux14/2 -> Mux1/16
  Demux14/4 -> Mux3/16
  Demux15/1 -> Mux/17
  Demux15/2 -> Mux1/17
  Demux15/3 -> Mux2/17
  Demux15/4 -> Mux3/17
  BitBasher/1 -> Scope/2, Mux1/1, Mux3/1, Mux2/1, Mux/1
  Gateway Out6/1 -> Mux5/2
  Gateway Out5/1 -> Mux5/1
  Gateway Out4/1 -> Mux4/2
  Gateway Out3/1 -> Mux4/1
  Mux4/1 -> block downconverter Scope/1
  Mux5/1 -> block downconverter Scope/2

== system CryoDetMultiChan_CMB/DspCore/FTA_Ch0/SixteenLineUDC 0/debug Scope ==
  note: Debug Demodulation
  demod : Inport
  freq : Inport  Port=2
  Complex to Magnitude-Angle : ComplexToMagnitudeAngle  Output=Magnitude
  Demux1 : Demux
  Gain : Gain  Gain=Fclk
  Gateway Out{1,3..6} (5 alike) : xbsIndex_r4/Gateway Out  inherit_from_input=off  hdl_port=off  rows=1  columns=1  UseAsDAC=off  DACChannel='1'  interface=None  automatic_assignment=on  address_offset=hex2dec('00')  intf_name=''  intf_description=''  timing_constraint=None  locs_specified=off  LOCs={}  io_standard={}  block_type=gatewayout
  Mux4 : Mux  Inputs=3
  Mux5 : Mux  Inputs=2
  Real-Imag to Complex : RealImagToComplex
  dbg block downconverter Scope : Scope  NumInputPorts=4
  wires:
  Gain/1 -> dbg block downconverter Scope/3
  Gateway Out1/1 -> Gain/1
  freq/1 -> Gateway Out1/1
  Real-Imag to Complex/1 -> Complex to Magnitude-Angle/1
  Complex to Magnitude-Angle/1 -> Mux4/3
  Mux5/1 -> dbg block downconverter Scope/2
  Mux4/1 -> dbg block downconverter Scope/1
  Gateway Out3/1 -> Real-Imag to Complex/2, Mux4/1
  Gateway Out4/1 -> Real-Imag to Complex/1, Mux4/2
  Gateway Out5/1 -> Mux5/1
  Gateway Out6/1 -> Mux5/2
  Demux1/4 -> Gateway Out6/1
  Demux1/3 -> Gateway Out5/1
  Demux1/2 -> Gateway Out4/1
  Demux1/1 -> Gateway Out3/1
  demod/1 -> Demux1/1
  [ch0_dF_latched] -> dbg block downconverter Scope/4
